simulink model "if_test"  (R2019a)
settings: Solver=VariableStepAuto  StartTime=0.0  StopTime=20  RelTol=1e-3
settings Model: Creator=asmialek  LastModifiedBy=asmialek

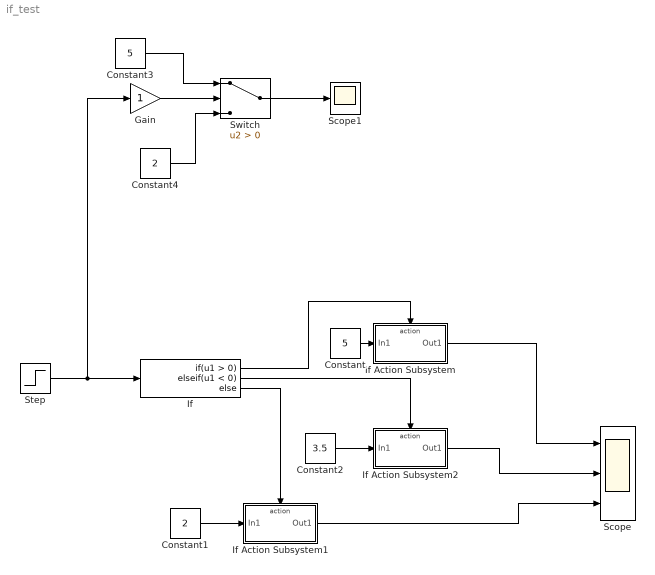
== system if_test ==
  Constant : Constant  Value=5
  Constant1 : Constant  Value=2
  Constant2 : Constant  Value=3.5
  Constant3 : Constant  Value=5
  Constant4 : Constant  Value=2
  Gain : Gain
  If : If  ElseIfExpressions=u1 < 0
  If Action Subsystem : Subsystem  TreatAsAtomicUnit=on
  If Action Subsystem1 : Subsystem  TreatAsAtomicUnit=on
  If Action Subsystem2 : Subsystem  TreatAsAtomicUnit=on
  Scope : Scope  NumInputPorts=3
  Scope1 : Scope
  Step : Step  Time=10  Before=-1  SampleTime=0
  Switch : Switch  Criteria=u2 > Threshold
  wires:
  Step/1 -> Gain/1, If/1
  If/3 -> If Action Subsystem1/Action
  If/1 -> If Action Subsystem/Action
  If Action Subsystem1/1(Out1) -> Scope/3
  If Action Subsystem/1(Out1) -> Scope/1
  Constant1/1 -> If Action Subsystem1/1(In1)
  Constant/1 -> If Action Subsystem/1(In1)
  If/2 -> If Action Subsystem2/Action
  Constant2/1 -> If Action Subsystem2/1(In1)
  If Action Subsystem2/1(Out1) -> Scope/2
  Constant3/1 -> Switch/1
  Constant4/1 -> Switch/3
  Switch/1 -> Scope1/1
  Gain/1 -> Switch/2

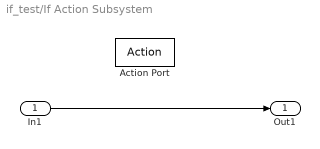
== system if_test/If Action Subsystem ==
  In1 : Inport
  Action Port : ActionPort  ActionPortLabel=if(u1 > 0)
  Out1 : Outport
  wires:
  In1/1 -> Out1/1

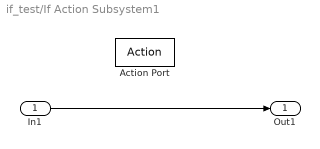
== system if_test/If Action Subsystem1 ==
  In1 : Inport
  Action Port : ActionPort  ActionPortLabel=else
  Out1 : Outport
  wires:
  In1/1 -> Out1/1

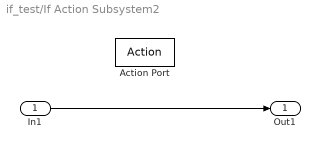
== system if_test/If Action Subsystem2 ==
  In1 : Inport
  Action Port : ActionPort  ActionPortLabel=elseif(u1 < 0)
  Out1 : Outport
  wires:
  In1/1 -> Out1/1
